simulink model "block_2ndorder_final"  (R2017b)
settings: Solver=VariableStepAuto  StartTime=0.0  StopTime=100  RelTol=1e-3
settings Model: Creator=Nick  LastModifiedBy=Nick

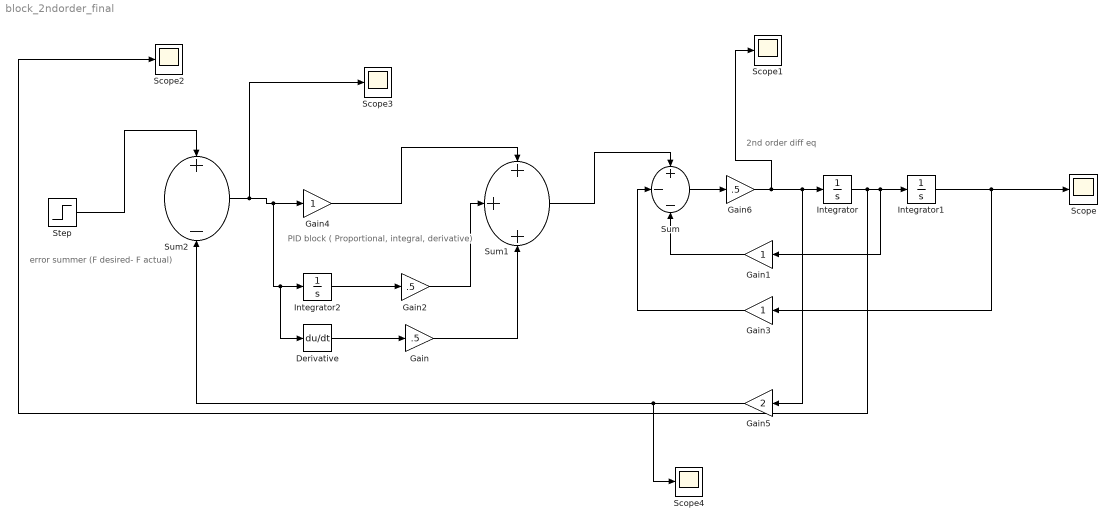
== system block_2ndorder_final ==
  note: 2nd order diff eq
  note: PID block ( Proportional, integral, derivative)
  note: error summer (F desired- F actual)
  Derivative : Derivative
  Gain : Gain  Gain=.5
  Gain1 : Gain
  Gain2 : Gain  Gain=.5
  Gain3 : Gain
  Gain4 : Gain
  Gain5 : Gain  Gain=2
  Gain6 : Gain  Gain=.5
  Integrator : Integrator
  Integrator1 : Integrator
  Integrator2 : Integrator
  Scope{,1..4} (5 alike) : Scope
  Step : Step  SampleTime=0
  Sum : Sum  Inputs=+--
  Sum1 : Sum  Inputs=+++
  Sum2 : Sum  Inputs=+-
  wires:
  Integrator/1 -> Scope2/1, Gain1/1, Integrator1/1
  Integrator1/1 -> Gain3/1, Scope/1
  Sum/1 -> Gain6/1
  Gain3/1 -> Sum/2
  Gain1/1 -> Sum/3
  Integrator2/1 -> Gain2/1
  Derivative/1 -> Gain/1
  Gain2/1 -> Sum1/2
  Gain/1 -> Sum1/3
  Gain4/1 -> Sum1/1
  Sum2/1 -> Scope3/1, Derivative/1, Integrator2/1, Gain4/1
  Gain5/1 -> Scope4/1, Sum2/2
  Gain6/1 -> Scope1/1, Gain5/1, Integrator/1
  Step/1 -> Sum2/1
  Sum1/1 -> Sum/1
